simulink model "NDI"  (R2022a)
settings: Solver=ode4  StartTime=0  StopTime=100  FixedStep=fcs.Ts  RelTol=1e-3
undefined symbols (not defined in the file or in its folder): Aactuator, ac, AeroCoeff, ControlAllocation, DUmax, DUmin, EngineTable, F, fcs, ft, g, hground, IC, kg, LandingGear, Light, m, MIL, Mode_deflection_aileron, Mode_deflection_elevator, Mode_deflection_rudder, Mode_deflection_TVC_y, Mode_deflection_TVC_z, N, Ninv_2nozzle, Ninv_no_nozzle, PIController, s, Sensor, sigbuilder_block, slug, state0, sysID_DAQ, sysID_OBES, Umax_2nozzle, Umax_no_nozzle, Umin_2nozzle, Umin_no_nozzle, WMM2020
libraries: aerolibconvert2 x31, slpidlib x11, simulink x6, sharedutil x4, aerolibatmos2 x3, aerolibwind2 x3, aerolibbdyn x3, aerolibgravity2 x2, sharedtransform x1
(part 2 of 13)

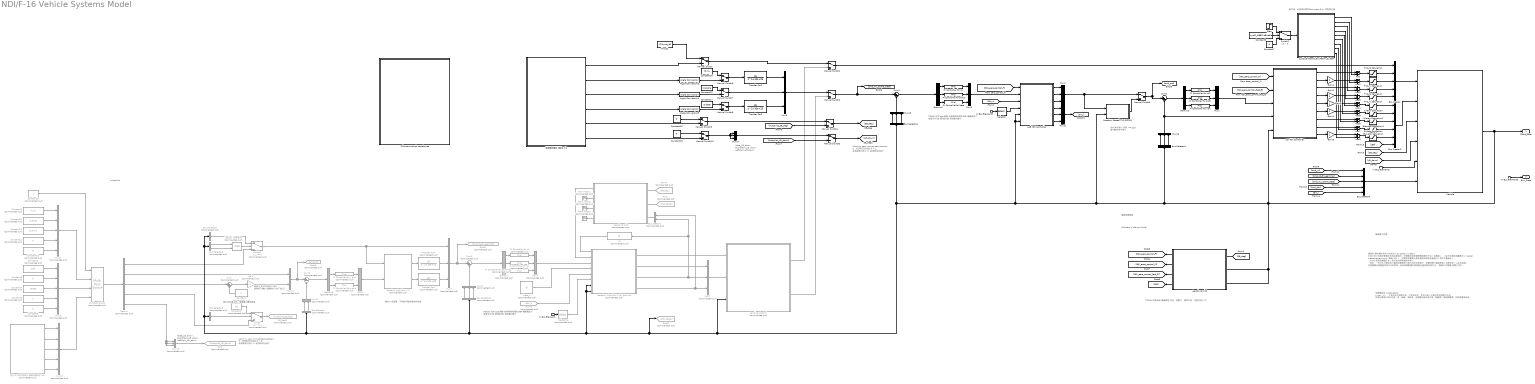
== system NDI/F-16 Vehicle Systems Model ==
  note: Onboard Airframe Model
  note: 高度 h_ft 命令是向上為正，
      | 要再乘-1轉成z座標命令(向下為正)
  note: Nose_LG_down
      | RightMain_LG_down
      | LeftMain_LG_down
  note: TODO: 改成local變數
      | 或者應該新增為OBM機載模型!?
      | 或者空中NDI跟地面NDI控制器分離!?
  note: 用於落地滑行
      | 速度 <= 220 會判斷為落地滑行
  note: 機載電子設備
  note: 全靜壓系統（pitot-static system），又稱為皮托靜壓系統、空速管系統，是飛行器上收集全壓與靜壓的系統，
      | 用來計算飛行時的空速、馬赫數、海拔等。全靜壓系統由皮托管、靜壓源、備用靜壓源、加熱裝置等組成。
  note: 傳統的 慣性導航系統(inertial navigation system (INS))至少包括計算機及含有加速度計、陀螺儀或其他運動傳感器的平台（或模組）。
      | INS包含慣性測量單元（Inertial measurement unit，簡稱 IMU ），該慣性測量單元具有角度和線性加速度計（用於位置變化）；
      | 一些IMU包括陀螺儀元件（用於保持絕對角度參考）。
      | 一般的，一個IMU內會裝有三軸的陀螺儀和三個方向的加速度計，測量物體三軸姿態角（或角速率）以及加速度。
      |
      | 在飛機顯示裝置變得現代化的同時，為其採集數據的感測器也變得更為現代化。
      | 傳統的 陀螺儀 被電子式的 航向姿態基準系統 （AHRS）與 大氣數據計算機 （ADC）所取代，
      | 在增加可靠性的同時也降低了成本、簡化了維護。
      | 此外， GPS 接收器也被整合進了玻璃駕駛艙之中。
  note: Landing gear normalized position
      | 0 : 起落架完全收起
      | 0 ~ 1: 起落架部分放下
      | 1: 起落架完全放下
  note: 拿掉!?
      | 先留著，不然配平點容易控制失敗
  note: 靜止在跑道上時，機身重心離地高度
  note: Autopilot
  note: Landing gear normalized position.
      | 0 : 起落架完全收起
      | 0 ~ 1: 起落架部分放下
      | 1: 起落架完全放下
  note: Nose_LG_down
      | RightMain_LG_down
      | LeftMain_LG_down
  note: TODO: 改成local變數
      | 或者應該新增為OBM機載模型!?
      | 或者空中NDI跟地面NDI控制器分離!?
  note: TODO: 改稱OBM機載模型
      | 內含：氣動力、標準大氣、地面作用力(?)
  note: 機載飛機模型
  note: 配平時，必須將此模塊Comment Out，否則會出錯
  In Bus Element1 : Inport  PortName=EnvData
  In Bus Element3 : Inport  PortName=EnvData
  In Bus Element2 : Inport  PortName=EnvData  Element=g
  In Bus Element : Inport  PortName=EnvData  Element=g
  Add{,1..8} (9 alike) : Sum
  Aerodynamic1 : Subsystem
  Aerodynamic2 : Subsystem  Commented=on
  Aileron Saturation : Saturate  UpperLimit=Aactuator.aileron.AngleLimitUpper  LowerLimit=Aactuator.aileron.AngleLimitLower
  Aileron Saturation1 : Saturate  UpperLimit=Aactuator.aileron.AngleLimitUpper  LowerLimit=Aactuator.aileron.AngleLimitLower
  Angle Conversion3 : aerolibconvert2/Angle Conversion  IU=deg  OU=rad
  Angle Conversion4 : aerolibconvert2/Angle Conversion  IU=deg  OU=rad
  Angle Conversion5 : aerolibconvert2/Angle Conversion  IU=deg  OU=rad
  Bus Creator : BusCreator  Inputs=5
  Bus Creator1 : BusCreator  Commented=on  Inputs=2
  Bus Creator2 : BusCreator  Inputs=6
  Bus Creator3 : BusCreator  Inputs=5
  Bus Selector : BusSelector  Commented=on  OutputSignals=epos,altitude
  Bus Selector1 : BusSelector  OutputSignals=p,q,r
  Bus Selector2 : BusSelector  Commented=on  OutputSignals=Vt
  Bus Selector3 : BusSelector  Commented=on  OutputSignals=Vt,chi,gamma
  Bus Selector4 : BusSelector  OutputSignals=mu,alpha,beta
  Bus Selector5 : BusSelector  Commented=on  OutputSignals=LGBus.Nose_WOW
  Bus Selector6 : BusSelector  Commented=on  OutputSignals=LGBus.RightMain_WOW,LGBus.LeftMain_WOW
  Constant{,3,5..6,12..13} (6 alike) : Constant  Commented=on  Value=0
  Constant1 : Constant  Commented=on  Value=60
  Constant10 : Constant  Commented=on  Value=IC.epos
  Constant11 : Constant  Commented=on  Value=IC.alt*-1
  Constant14 : Constant  Commented=on
  Constant15 : Constant  Value=IC.alpha
  Constant16 : Constant  Value=IC.mu
  Constant17 : Constant  Value=IC.beta
  Constant18 : Constant  Value=0
  Constant19 : Constant  Value=0
  Constant2 : Constant  Commented=on  Value=450
  Constant4 : Constant  Commented=on  Value=10000
  Constant7 : Constant  Value=0
  Constant8 : Constant  Value=sysID_OBES.isEnable
  Constant9 : Constant  Commented=on  Value=IC.Vt
  Demux : Demux  Commented=on  Outputs=5
  Demux1 : Demux  Commented=on  Outputs=3
  Demux3 : Demux  Outputs=3
  Demux5 : Demux  Commented=on  Outputs=2
  Demux6 : Demux  Outputs=3
  Elevator Saturation : Saturate  UpperLimit=Aactuator.elevator.AngleLimitUpper  LowerLimit=Aactuator.elevator.AngleLimitLower
  Elevator Saturation1 : Saturate  UpperLimit=Aactuator.elevator.AngleLimitUpper  LowerLimit=Aactuator.elevator.AngleLimitLower
  From : From  Commented=on  GotoTag=PlantData
  From4 : From  Commented=on  GotoTag=SB_deg
  From5 : From  Commented=on  GotoTag=LGxyz  TagVisibility=global
      settings: CloseFcn=tagdialog Close
  Gain : Gain  Commented=on  Gain=-1
  Gain{1..5} (5 alike) : Gain
  Goto : Goto  Commented=on  GotoTag=Autopilot_LG_down
  Goto1 : Goto  Commented=on  GotoTag=cmd_Vt_chi_gamma
  Goto2 : Goto  Commented=on  GotoTag=PlantData
  Goto8 : Goto  Commented=on  GotoTag=cmd_yz
  IC : InitialCondition  Commented=on  Value=IC.alpha
  Iteration Algorithm V chi gamma : Subsystem  Commented=on
  Iteration Algorithm Y Z : Subsystem  Commented=on
  Landing_Control : Subsystem  Commented=on
  Logical Operator : Logic  Commented=on  AllPortsSameDT=off  OutDataTypeStr=boolean
  Manual Switch{,1..10} (11 alike) : ManualSwitch
  Multiport Switch : MultiPortSwitch  Commented=on  SaturateOnIntegerOverflow=off  InputSameDT=off
  Mux{1..2,5..6,11,14,16,18} (8 alike) : Mux  Inputs=3
  Mux10 : Mux  Commented=on  Inputs=2
  Mux12 : Mux  Commented=on  Inputs=2
  Mux{3..4,7,13,17} (5 alike) : Mux  Commented=on  Inputs=3
  Mux15 : Mux  Commented=on  Inputs=5
  Mux19 : Mux  Commented=on  Inputs=5
  Mux8 : Mux  Commented=on  Inputs=5
  Mux9 : Mux  Commented=on  Inputs=2
  PI Controller for Vt : slpidlib/PID Controller  Commented=on  Controller=PI  Form=Parallel  TimeDomain=Continuous-time  UseExternalTs=off  SampleTime=-1  IntegratorMethod=Forward Euler  FilterMethod=Forward Euler  ControllerParametersSource=internal  P=PIController.Vt.P  I=PIController.Vt.I  UseKiTs=off  D=0  N=100  UseFilter=on  TunerSelectOption=Transfer Function Based (PID Tuner App)  InitialConditionSource=internal  InitialConditionForIntegrator=0  InitialConditionForFilter=0  DifferentiatorICPrevScaledInput=0  ExternalReset=none  TrackingMode=off  Kt=1  LimitOutput=off  SatLimitsSource=internal  UpperSaturationLimit=inf  LowerSaturationLimit=-inf  LinearizeAsGain=on  AntiWindupMode=none  Kb=1  POutMin=[]  POutMax=[]  IOutMin=[]  IOutMax=[]  DOutMin=[]  DOutMax=[]  NOutMin=[]  NOutMax=[]  SumOutMin=[]  SumOutMax=[]  SaturationOutMin=[]  SaturationOutMax=[]  PParamMin=[]  PParamMax=[]  IParamMin=[]  IParamMax=[]  DParamMin=[]  DParamMax=[]  NParamMin=[]  NParamMax=[]  KbParamMin=[]  KbParamMax=[]  KtParamMin=[]  KtParamMax=[]  KbOutMin=[]  KbOutMax=[]  KtOutMin=[]  KtOutMax=[]  IntegratorOutMin=[]  IntegratorOutMax=[]  FilterOutMin=[]  FilterOutMax=[]  SumI1OutMin=[]  SumI1OutMax=[]  SumI2OutMin=[]  SumI2OutMax=[]  SumI3OutMin=[]  SumI3OutMax=[]  SumI4OutMin=[]  SumI4OutMax=[]  SumDOutMin=[]  SumDOutMax=[]  DifferentiatorOutMin=[]  DifferentiatorOutMax=[]  FilterDiffOutCoefMin=[]  FilterDiffOutCoefMax=[]  ReciprocalOutMin=[]  ReciprocalOutMax=[]  SumDenOutMin=[]  SumDenOutMax=[]  SumNumOutMin=[]  SumNumOutMax=[]  DivideOutMin=[]  DivideOutMax=[]  UdiffTsProdOutMin=[]  UdiffTsProdOutMax=[]  NTsProdOutMin=[]  NTsProdOutMax=[]  UintegralTsProdOutMin=[]  UintegralTsProdOutMax=[]  UngainTsProdOutMin=[]  UngainTsProdOutMax=[]  IntegratorContinuousStateAttributes=''  IntegratorStateMustResolveToSignalObject=off  IntegratorRTWStateStorageClass=Auto  FilterContinuousStateAttributes=''  FilterStateMustResolveToSignalObject=off  FilterRTWStateStorageClass=Auto  ParallelPVariant=InternalParameters  IdealPVariant=Disabled  IVariant=InternalParameters  DVariant=Disabled  IntegratorVariant=Continuous  SatVariant=Disabled  AWVariant=Passthrough  PCopyVariant=Disabled  TRVariant=Disabled  FdbkBlocksVariant=Forward  IdealPFdbkVariant=Disabled  SatFdbkVariant=Disabled  DerivativeFilterVariant=Disabled  NVariant=Disabled  NCopyVariant=Disabled_SignalSpec  FilterICVariant=Disabled  IntegratorICVariant=InternalICs  ExternalResetVariant=Disabled  TRSumVariant=Passthrough  SumFdbkVariant=Disabled  SumVariant=Sum_PI  TsampFilterVariant=InternalTs  TsampNgainVariant=Passthrough  TsampIntegralVariant=Passthrough  ExternalSaturationOutDataTypeStr=Inherit: Same as second input  aMode=0
  PI Controller for alpha : slpidlib/PID Controller  Controller=PI  Form=Parallel  TimeDomain=Continuous-time  UseExternalTs=off  SampleTime=-1  IntegratorMethod=Forward Euler  FilterMethod=Forward Euler  ControllerParametersSource=internal  P=PIController.alpha.P  I=PIController.alpha.I  UseKiTs=off  D=0  N=100  UseFilter=on  TunerSelectOption=Transfer Function Based (PID Tuner App)  InitialConditionSource=internal  InitialConditionForIntegrator=0  InitialConditionForFilter=0  DifferentiatorICPrevScaledInput=0  ExternalReset=none  TrackingMode=off  Kt=1  LimitOutput=off  SatLimitsSource=internal  UpperSaturationLimit=inf  LowerSaturationLimit=-inf  LinearizeAsGain=on  AntiWindupMode=none  Kb=1  POutMin=[]  POutMax=[]  IOutMin=[]  IOutMax=[]  DOutMin=[]  DOutMax=[]  NOutMin=[]  NOutMax=[]  SumOutMin=[]  SumOutMax=[]  SaturationOutMin=[]  SaturationOutMax=[]  PParamMin=[]  PParamMax=[]  IParamMin=[]  IParamMax=[]  DParamMin=[]  DParamMax=[]  NParamMin=[]  NParamMax=[]  KbParamMin=[]  KbParamMax=[]  KtParamMin=[]  KtParamMax=[]  KbOutMin=[]  KbOutMax=[]  KtOutMin=[]  KtOutMax=[]  IntegratorOutMin=[]  IntegratorOutMax=[]  FilterOutMin=[]  FilterOutMax=[]  SumI1OutMin=[]  SumI1OutMax=[]  SumI2OutMin=[]  SumI2OutMax=[]  SumI3OutMin=[]  SumI3OutMax=[]  SumI4OutMin=[]  SumI4OutMax=[]  SumDOutMin=[]  SumDOutMax=[]  DifferentiatorOutMin=[]  DifferentiatorOutMax=[]  FilterDiffOutCoefMin=[]  FilterDiffOutCoefMax=[]  ReciprocalOutMin=[]  ReciprocalOutMax=[]  SumDenOutMin=[]  SumDenOutMax=[]  SumNumOutMin=[]  SumNumOutMax=[]  DivideOutMin=[]  DivideOutMax=[]  UdiffTsProdOutMin=[]  UdiffTsProdOutMax=[]  NTsProdOutMin=[]  NTsProdOutMax=[]  UintegralTsProdOutMin=[]  UintegralTsProdOutMax=[]  UngainTsProdOutMin=[]  UngainTsProdOutMax=[]  IntegratorContinuousStateAttributes=''  IntegratorStateMustResolveToSignalObject=off  IntegratorRTWStateStorageClass=Auto  FilterContinuousStateAttributes=''  FilterStateMustResolveToSignalObject=off  FilterRTWStateStorageClass=Auto  ParallelPVariant=InternalParameters  IdealPVariant=Disabled  IVariant=InternalParameters  DVariant=Disabled  IntegratorVariant=Continuous  SatVariant=Disabled  AWVariant=Passthrough  PCopyVariant=Disabled  TRVariant=Disabled  FdbkBlocksVariant=Forward  IdealPFdbkVariant=Disabled  SatFdbkVariant=Disabled  DerivativeFilterVariant=Disabled  NVariant=Disabled  NCopyVariant=Disabled_SignalSpec  FilterICVariant=Disabled  IntegratorICVariant=InternalICs  ExternalResetVariant=Disabled  TRSumVariant=Passthrough  SumFdbkVariant=Disabled  SumVariant=Sum_PI  TsampFilterVariant=InternalTs  TsampNgainVariant=Passthrough  TsampIntegralVariant=Passthrough  ExternalSaturationOutDataTypeStr=Inherit: Same as second input  aMode=0
  PI Controller for beta : slpidlib/PID Controller  Controller=PI  Form=Parallel  TimeDomain=Continuous-time  UseExternalTs=off  SampleTime=-1  IntegratorMethod=Forward Euler  FilterMethod=Forward Euler  ControllerParametersSource=internal  P=PIController.beta.P  I=PIController.beta.I  UseKiTs=off  D=0  N=100  UseFilter=on  TunerSelectOption=Transfer Function Based (PID Tuner App)  InitialConditionSource=internal  InitialConditionForIntegrator=0  InitialConditionForFilter=0  DifferentiatorICPrevScaledInput=0  ExternalReset=none  TrackingMode=off  Kt=1  LimitOutput=off  SatLimitsSource=internal  UpperSaturationLimit=inf  LowerSaturationLimit=-inf  LinearizeAsGain=on  AntiWindupMode=none  Kb=1  POutMin=[]  POutMax=[]  IOutMin=[]  IOutMax=[]  DOutMin=[]  DOutMax=[]  NOutMin=[]  NOutMax=[]  SumOutMin=[]  SumOutMax=[]  SaturationOutMin=[]  SaturationOutMax=[]  PParamMin=[]  PParamMax=[]  IParamMin=[]  IParamMax=[]  DParamMin=[]  DParamMax=[]  NParamMin=[]  NParamMax=[]  KbParamMin=[]  KbParamMax=[]  KtParamMin=[]  KtParamMax=[]  KbOutMin=[]  KbOutMax=[]  KtOutMin=[]  KtOutMax=[]  IntegratorOutMin=[]  IntegratorOutMax=[]  FilterOutMin=[]  FilterOutMax=[]  SumI1OutMin=[]  SumI1OutMax=[]  SumI2OutMin=[]  SumI2OutMax=[]  SumI3OutMin=[]  SumI3OutMax=[]  SumI4OutMin=[]  SumI4OutMax=[]  SumDOutMin=[]  SumDOutMax=[]  DifferentiatorOutMin=[]  DifferentiatorOutMax=[]  FilterDiffOutCoefMin=[]  FilterDiffOutCoefMax=[]  ReciprocalOutMin=[]  ReciprocalOutMax=[]  SumDenOutMin=[]  SumDenOutMax=[]  SumNumOutMin=[]  SumNumOutMax=[]  DivideOutMin=[]  DivideOutMax=[]  UdiffTsProdOutMin=[]  UdiffTsProdOutMax=[]  NTsProdOutMin=[]  NTsProdOutMax=[]  UintegralTsProdOutMin=[]  UintegralTsProdOutMax=[]  UngainTsProdOutMin=[]  UngainTsProdOutMax=[]  IntegratorContinuousStateAttributes=''  IntegratorStateMustResolveToSignalObject=off  IntegratorRTWStateStorageClass=Auto  FilterContinuousStateAttributes=''  FilterStateMustResolveToSignalObject=off  FilterRTWStateStorageClass=Auto  ParallelPVariant=InternalParameters  IdealPVariant=Disabled  IVariant=InternalParameters  DVariant=Disabled  IntegratorVariant=Continuous  SatVariant=Disabled  AWVariant=Passthrough  PCopyVariant=Disabled  TRVariant=Disabled  FdbkBlocksVariant=Forward  IdealPFdbkVariant=Disabled  SatFdbkVariant=Disabled  DerivativeFilterVariant=Disabled  NVariant=Disabled  NCopyVariant=Disabled_SignalSpec  FilterICVariant=Disabled  IntegratorICVariant=InternalICs  ExternalResetVariant=Disabled  TRSumVariant=Passthrough  SumFdbkVariant=Disabled  SumVariant=Sum_PI  TsampFilterVariant=InternalTs  TsampNgainVariant=Passthrough  TsampIntegralVariant=Passthrough  ExternalSaturationOutDataTypeStr=Inherit: Same as second input  aMode=0
  PI Controller for chi : slpidlib/PID Controller  Commented=on  Controller=PI  Form=Parallel  TimeDomain=Continuous-time  UseExternalTs=off  SampleTime=-1  IntegratorMethod=Forward Euler  FilterMethod=Forward Euler  ControllerParametersSource=internal  P=PIController.chi.P  I=PIController.chi.I  UseKiTs=off  D=0  N=100  UseFilter=on  TunerSelectOption=Transfer Function Based (PID Tuner App)  InitialConditionSource=internal  InitialConditionForIntegrator=0  InitialConditionForFilter=0  DifferentiatorICPrevScaledInput=0  ExternalReset=none  TrackingMode=off  Kt=1  LimitOutput=off  SatLimitsSource=internal  UpperSaturationLimit=inf  LowerSaturationLimit=-inf  LinearizeAsGain=on  AntiWindupMode=none  Kb=1  POutMin=[]  POutMax=[]  IOutMin=[]  IOutMax=[]  DOutMin=[]  DOutMax=[]  NOutMin=[]  NOutMax=[]  SumOutMin=[]  SumOutMax=[]  SaturationOutMin=[]  SaturationOutMax=[]  PParamMin=[]  PParamMax=[]  IParamMin=[]  IParamMax=[]  DParamMin=[]  DParamMax=[]  NParamMin=[]  NParamMax=[]  KbParamMin=[]  KbParamMax=[]  KtParamMin=[]  KtParamMax=[]  KbOutMin=[]  KbOutMax=[]  KtOutMin=[]  KtOutMax=[]  IntegratorOutMin=[]  IntegratorOutMax=[]  FilterOutMin=[]  FilterOutMax=[]  SumI1OutMin=[]  SumI1OutMax=[]  SumI2OutMin=[]  SumI2OutMax=[]  SumI3OutMin=[]  SumI3OutMax=[]  SumI4OutMin=[]  SumI4OutMax=[]  SumDOutMin=[]  SumDOutMax=[]  DifferentiatorOutMin=[]  DifferentiatorOutMax=[]  FilterDiffOutCoefMin=[]  FilterDiffOutCoefMax=[]  ReciprocalOutMin=[]  ReciprocalOutMax=[]  SumDenOutMin=[]  SumDenOutMax=[]  SumNumOutMin=[]  SumNumOutMax=[]  DivideOutMin=[]  DivideOutMax=[]  UdiffTsProdOutMin=[]  UdiffTsProdOutMax=[]  NTsProdOutMin=[]  NTsProdOutMax=[]  UintegralTsProdOutMin=[]  UintegralTsProdOutMax=[]  UngainTsProdOutMin=[]  UngainTsProdOutMax=[]  IntegratorContinuousStateAttributes=''  IntegratorStateMustResolveToSignalObject=off  IntegratorRTWStateStorageClass=Auto  FilterContinuousStateAttributes=''  FilterStateMustResolveToSignalObject=off  FilterRTWStateStorageClass=Auto  ParallelPVariant=InternalParameters  IdealPVariant=Disabled  IVariant=InternalParameters  DVariant=Disabled  IntegratorVariant=Continuous  SatVariant=Disabled  AWVariant=Passthrough  PCopyVariant=Disabled  TRVariant=Disabled  FdbkBlocksVariant=Forward  IdealPFdbkVariant=Disabled  SatFdbkVariant=Disabled  DerivativeFilterVariant=Disabled  NVariant=Disabled  NCopyVariant=Disabled_SignalSpec  FilterICVariant=Disabled  IntegratorICVariant=InternalICs  ExternalResetVariant=Disabled  TRSumVariant=Passthrough  SumFdbkVariant=Disabled  SumVariant=Sum_PI  TsampFilterVariant=InternalTs  TsampNgainVariant=Passthrough  TsampIntegralVariant=Passthrough  ExternalSaturationOutDataTypeStr=Inherit: Same as second input  aMode=0
  PI Controller for gamma : slpidlib/PID Controller  Commented=on  Controller=PI  Form=Parallel  TimeDomain=Continuous-time  UseExternalTs=off  SampleTime=-1  IntegratorMethod=Forward Euler  FilterMethod=Forward Euler  ControllerParametersSource=internal  P=PIController.gamma.P  I=PIController.gamma.I  UseKiTs=off  D=0  N=100  UseFilter=on  TunerSelectOption=Transfer Function Based (PID Tuner App)  InitialConditionSource=internal  InitialConditionForIntegrator=0  InitialConditionForFilter=0  DifferentiatorICPrevScaledInput=0  ExternalReset=none  TrackingMode=off  Kt=1  LimitOutput=off  SatLimitsSource=internal  UpperSaturationLimit=inf  LowerSaturationLimit=-inf  LinearizeAsGain=on  AntiWindupMode=none  Kb=1  POutMin=[]  POutMax=[]  IOutMin=[]  IOutMax=[]  DOutMin=[]  DOutMax=[]  NOutMin=[]  NOutMax=[]  SumOutMin=[]  SumOutMax=[]  SaturationOutMin=[]  SaturationOutMax=[]  PParamMin=[]  PParamMax=[]  IParamMin=[]  IParamMax=[]  DParamMin=[]  DParamMax=[]  NParamMin=[]  NParamMax=[]  KbParamMin=[]  KbParamMax=[]  KtParamMin=[]  KtParamMax=[]  KbOutMin=[]  KbOutMax=[]  KtOutMin=[]  KtOutMax=[]  IntegratorOutMin=[]  IntegratorOutMax=[]  FilterOutMin=[]  FilterOutMax=[]  SumI1OutMin=[]  SumI1OutMax=[]  SumI2OutMin=[]  SumI2OutMax=[]  SumI3OutMin=[]  SumI3OutMax=[]  SumI4OutMin=[]  SumI4OutMax=[]  SumDOutMin=[]  SumDOutMax=[]  DifferentiatorOutMin=[]  DifferentiatorOutMax=[]  FilterDiffOutCoefMin=[]  FilterDiffOutCoefMax=[]  ReciprocalOutMin=[]  ReciprocalOutMax=[]  SumDenOutMin=[]  SumDenOutMax=[]  SumNumOutMin=[]  SumNumOutMax=[]  DivideOutMin=[]  DivideOutMax=[]  UdiffTsProdOutMin=[]  UdiffTsProdOutMax=[]  NTsProdOutMin=[]  NTsProdOutMax=[]  UintegralTsProdOutMin=[]  UintegralTsProdOutMax=[]  UngainTsProdOutMin=[]  UngainTsProdOutMax=[]  IntegratorContinuousStateAttributes=''  IntegratorStateMustResolveToSignalObject=off  IntegratorRTWStateStorageClass=Auto  FilterContinuousStateAttributes=''  FilterStateMustResolveToSignalObject=off  FilterRTWStateStorageClass=Auto  ParallelPVariant=InternalParameters  IdealPVariant=Disabled  IVariant=InternalParameters  DVariant=Disabled  IntegratorVariant=Continuous  SatVariant=Disabled  AWVariant=Passthrough  PCopyVariant=Disabled  TRVariant=Disabled  FdbkBlocksVariant=Forward  IdealPFdbkVariant=Disabled  SatFdbkVariant=Disabled  DerivativeFilterVariant=Disabled  NVariant=Disabled  NCopyVariant=Disabled_SignalSpec  FilterICVariant=Disabled  IntegratorICVariant=InternalICs  ExternalResetVariant=Disabled  TRSumVariant=Passthrough  SumFdbkVariant=Disabled  SumVariant=Sum_PI  TsampFilterVariant=InternalTs  TsampNgainVariant=Passthrough  TsampIntegralVariant=Passthrough  ExternalSaturationOutDataTypeStr=Inherit: Same as second input  aMode=0
  PI Controller for mu : slpidlib/PID Controller  Controller=PI  Form=Parallel  TimeDomain=Continuous-time  UseExternalTs=off  SampleTime=-1  IntegratorMethod=Forward Euler  FilterMethod=Forward Euler  ControllerParametersSource=internal  P=PIController.mu.P  I=PIController.mu.I  UseKiTs=off  D=0  N=100  UseFilter=on  TunerSelectOption=Transfer Function Based (PID Tuner App)  InitialConditionSource=internal  InitialConditionForIntegrator=0  InitialConditionForFilter=0  DifferentiatorICPrevScaledInput=0  ExternalReset=none  TrackingMode=off  Kt=1  LimitOutput=off  SatLimitsSource=internal  UpperSaturationLimit=inf  LowerSaturationLimit=-inf  LinearizeAsGain=on  AntiWindupMode=none  Kb=1  POutMin=[]  POutMax=[]  IOutMin=[]  IOutMax=[]  DOutMin=[]  DOutMax=[]  NOutMin=[]  NOutMax=[]  SumOutMin=[]  SumOutMax=[]  SaturationOutMin=[]  SaturationOutMax=[]  PParamMin=[]  PParamMax=[]  IParamMin=[]  IParamMax=[]  DParamMin=[]  DParamMax=[]  NParamMin=[]  NParamMax=[]  KbParamMin=[]  KbParamMax=[]  KtParamMin=[]  KtParamMax=[]  KbOutMin=[]  KbOutMax=[]  KtOutMin=[]  KtOutMax=[]  IntegratorOutMin=[]  IntegratorOutMax=[]  FilterOutMin=[]  FilterOutMax=[]  SumI1OutMin=[]  SumI1OutMax=[]  SumI2OutMin=[]  SumI2OutMax=[]  SumI3OutMin=[]  SumI3OutMax=[]  SumI4OutMin=[]  SumI4OutMax=[]  SumDOutMin=[]  SumDOutMax=[]  DifferentiatorOutMin=[]  DifferentiatorOutMax=[]  FilterDiffOutCoefMin=[]  FilterDiffOutCoefMax=[]  ReciprocalOutMin=[]  ReciprocalOutMax=[]  SumDenOutMin=[]  SumDenOutMax=[]  SumNumOutMin=[]  SumNumOutMax=[]  DivideOutMin=[]  DivideOutMax=[]  UdiffTsProdOutMin=[]  UdiffTsProdOutMax=[]  NTsProdOutMin=[]  NTsProdOutMax=[]  UintegralTsProdOutMin=[]  UintegralTsProdOutMax=[]  UngainTsProdOutMin=[]  UngainTsProdOutMax=[]  IntegratorContinuousStateAttributes=''  IntegratorStateMustResolveToSignalObject=off  IntegratorRTWStateStorageClass=Auto  FilterContinuousStateAttributes=''  FilterStateMustResolveToSignalObject=off  FilterRTWStateStorageClass=Auto  ParallelPVariant=InternalParameters  IdealPVariant=Disabled  IVariant=InternalParameters  DVariant=Disabled  IntegratorVariant=Continuous  SatVariant=Disabled  AWVariant=Passthrough  PCopyVariant=Disabled  TRVariant=Disabled  FdbkBlocksVariant=Forward  IdealPFdbkVariant=Disabled  SatFdbkVariant=Disabled  DerivativeFilterVariant=Disabled  NVariant=Disabled  NCopyVariant=Disabled_SignalSpec  FilterICVariant=Disabled  IntegratorICVariant=InternalICs  ExternalResetVariant=Disabled  TRSumVariant=Passthrough  SumFdbkVariant=Disabled  SumVariant=Sum_PI  TsampFilterVariant=InternalTs  TsampNgainVariant=Passthrough  TsampIntegralVariant=Passthrough  ExternalSaturationOutDataTypeStr=Inherit: Same as second input  aMode=0
  PI Controller for pitch : slpidlib/PID Controller  Controller=PI  Form=Parallel  TimeDomain=Continuous-time  UseExternalTs=off  SampleTime=-1  IntegratorMethod=Forward Euler  FilterMethod=Forward Euler  ControllerParametersSource=internal  P=PIController.q.P  I=PIController.q.I  UseKiTs=off  D=0  N=100  UseFilter=on  TunerSelectOption=Transfer Function Based (PID Tuner App)  InitialConditionSource=internal  InitialConditionForIntegrator=0  InitialConditionForFilter=0  DifferentiatorICPrevScaledInput=0  ExternalReset=none  TrackingMode=off  Kt=1  LimitOutput=off  SatLimitsSource=internal  UpperSaturationLimit=inf  LowerSaturationLimit=-inf  LinearizeAsGain=on  AntiWindupMode=none  Kb=1  POutMin=[]  POutMax=[]  IOutMin=[]  IOutMax=[]  DOutMin=[]  DOutMax=[]  NOutMin=[]  NOutMax=[]  SumOutMin=[]  SumOutMax=[]  SaturationOutMin=[]  SaturationOutMax=[]  PParamMin=[]  PParamMax=[]  IParamMin=[]  IParamMax=[]  DParamMin=[]  DParamMax=[]  NParamMin=[]  NParamMax=[]  KbParamMin=[]  KbParamMax=[]  KtParamMin=[]  KtParamMax=[]  KbOutMin=[]  KbOutMax=[]  KtOutMin=[]  KtOutMax=[]  IntegratorOutMin=[]  IntegratorOutMax=[]  FilterOutMin=[]  FilterOutMax=[]  SumI1OutMin=[]  SumI1OutMax=[]  SumI2OutMin=[]  SumI2OutMax=[]  SumI3OutMin=[]  SumI3OutMax=[]  SumI4OutMin=[]  SumI4OutMax=[]  SumDOutMin=[]  SumDOutMax=[]  DifferentiatorOutMin=[]  DifferentiatorOutMax=[]  FilterDiffOutCoefMin=[]  FilterDiffOutCoefMax=[]  ReciprocalOutMin=[]  ReciprocalOutMax=[]  SumDenOutMin=[]  SumDenOutMax=[]  SumNumOutMin=[]  SumNumOutMax=[]  DivideOutMin=[]  DivideOutMax=[]  UdiffTsProdOutMin=[]  UdiffTsProdOutMax=[]  NTsProdOutMin=[]  NTsProdOutMax=[]  UintegralTsProdOutMin=[]  UintegralTsProdOutMax=[]  UngainTsProdOutMin=[]  UngainTsProdOutMax=[]  IntegratorContinuousStateAttributes=''  IntegratorStateMustResolveToSignalObject=off  IntegratorRTWStateStorageClass=Auto  FilterContinuousStateAttributes=''  FilterStateMustResolveToSignalObject=off  FilterRTWStateStorageClass=Auto  ParallelPVariant=InternalParameters  IdealPVariant=Disabled  IVariant=InternalParameters  DVariant=Disabled  IntegratorVariant=Continuous  SatVariant=Disabled  AWVariant=Passthrough  PCopyVariant=Disabled  TRVariant=Disabled  FdbkBlocksVariant=Forward  IdealPFdbkVariant=Disabled  SatFdbkVariant=Disabled  DerivativeFilterVariant=Disabled  NVariant=Disabled  NCopyVariant=Disabled_SignalSpec  FilterICVariant=Disabled  IntegratorICVariant=InternalICs  ExternalResetVariant=Disabled  TRSumVariant=Passthrough  SumFdbkVariant=Disabled  SumVariant=Sum_PI  TsampFilterVariant=InternalTs  TsampNgainVariant=Passthrough  TsampIntegralVariant=Passthrough  ExternalSaturationOutDataTypeStr=Inherit: Same as second input  aMode=0
  PI Controller for roll : slpidlib/PID Controller  Controller=PI  Form=Parallel  TimeDomain=Continuous-time  UseExternalTs=off  SampleTime=-1  IntegratorMethod=Forward Euler  FilterMethod=Forward Euler  ControllerParametersSource=internal  P=PIController.p.P  I=PIController.p.I  UseKiTs=off  D=0  N=100  UseFilter=on  TunerSelectOption=Transfer Function Based (PID Tuner App)  InitialConditionSource=internal  InitialConditionForIntegrator=0  InitialConditionForFilter=0  DifferentiatorICPrevScaledInput=0  ExternalReset=none  TrackingMode=off  Kt=1  LimitOutput=off  SatLimitsSource=internal  UpperSaturationLimit=inf  LowerSaturationLimit=-inf  LinearizeAsGain=on  AntiWindupMode=none  Kb=1  POutMin=[]  POutMax=[]  IOutMin=[]  IOutMax=[]  DOutMin=[]  DOutMax=[]  NOutMin=[]  NOutMax=[]  SumOutMin=[]  SumOutMax=[]  SaturationOutMin=[]  SaturationOutMax=[]  PParamMin=[]  PParamMax=[]  IParamMin=[]  IParamMax=[]  DParamMin=[]  DParamMax=[]  NParamMin=[]  NParamMax=[]  KbParamMin=[]  KbParamMax=[]  KtParamMin=[]  KtParamMax=[]  KbOutMin=[]  KbOutMax=[]  KtOutMin=[]  KtOutMax=[]  IntegratorOutMin=[]  IntegratorOutMax=[]  FilterOutMin=[]  FilterOutMax=[]  SumI1OutMin=[]  SumI1OutMax=[]  SumI2OutMin=[]  SumI2OutMax=[]  SumI3OutMin=[]  SumI3OutMax=[]  SumI4OutMin=[]  SumI4OutMax=[]  SumDOutMin=[]  SumDOutMax=[]  DifferentiatorOutMin=[]  DifferentiatorOutMax=[]  FilterDiffOutCoefMin=[]  FilterDiffOutCoefMax=[]  ReciprocalOutMin=[]  ReciprocalOutMax=[]  SumDenOutMin=[]  SumDenOutMax=[]  SumNumOutMin=[]  SumNumOutMax=[]  DivideOutMin=[]  DivideOutMax=[]  UdiffTsProdOutMin=[]  UdiffTsProdOutMax=[]  NTsProdOutMin=[]  NTsProdOutMax=[]  UintegralTsProdOutMin=[]  UintegralTsProdOutMax=[]  UngainTsProdOutMin=[]  UngainTsProdOutMax=[]  IntegratorContinuousStateAttributes=''  IntegratorStateMustResolveToSignalObject=off  IntegratorRTWStateStorageClass=Auto  FilterContinuousStateAttributes=''  FilterStateMustResolveToSignalObject=off  FilterRTWStateStorageClass=Auto  ParallelPVariant=InternalParameters  IdealPVariant=Disabled  IVariant=InternalParameters  DVariant=Disabled  IntegratorVariant=Continuous  SatVariant=Disabled  AWVariant=Passthrough  PCopyVariant=Disabled  TRVariant=Disabled  FdbkBlocksVariant=Forward  IdealPFdbkVariant=Disabled  SatFdbkVariant=Disabled  DerivativeFilterVariant=Disabled  NVariant=Disabled  NCopyVariant=Disabled_SignalSpec  FilterICVariant=Disabled  IntegratorICVariant=InternalICs  ExternalResetVariant=Disabled  TRSumVariant=Passthrough  SumFdbkVariant=Disabled  SumVariant=Sum_PI  TsampFilterVariant=InternalTs  TsampNgainVariant=Passthrough  TsampIntegralVariant=Passthrough  ExternalSaturationOutDataTypeStr=Inherit: Same as second input  aMode=0
  PI Controller for y axis : slpidlib/PID Controller  Commented=on  Controller=PI  Form=Parallel  TimeDomain=Continuous-time  UseExternalTs=off  SampleTime=-1  IntegratorMethod=Forward Euler  FilterMethod=Forward Euler  ControllerParametersSource=internal  P=PIController.y.P  I=PIController.y.I  UseKiTs=off  D=PIController.y.D  N=10  UseFilter=on  TunerSelectOption=Transfer Function Based (PID Tuner App)  InitialConditionSource=internal  InitialConditionForIntegrator=0  InitialConditionForFilter=0  DifferentiatorICPrevScaledInput=0  ExternalReset=none  TrackingMode=off  Kt=1  LimitOutput=off  SatLimitsSource=internal  UpperSaturationLimit=inf  LowerSaturationLimit=-inf  LinearizeAsGain=on  AntiWindupMode=none  Kb=1  POutMin=[]  POutMax=[]  IOutMin=[]  IOutMax=[]  DOutMin=[]  DOutMax=[]  NOutMin=[]  NOutMax=[]  SumOutMin=[]  SumOutMax=[]  SaturationOutMin=[]  SaturationOutMax=[]  PParamMin=[]  PParamMax=[]  IParamMin=[]  IParamMax=[]  DParamMin=[]  DParamMax=[]  NParamMin=[]  NParamMax=[]  KbParamMin=[]  KbParamMax=[]  KtParamMin=[]  KtParamMax=[]  KbOutMin=[]  KbOutMax=[]  KtOutMin=[]  KtOutMax=[]  IntegratorOutMin=[]  IntegratorOutMax=[]  FilterOutMin=[]  FilterOutMax=[]  SumI1OutMin=[]  SumI1OutMax=[]  SumI2OutMin=[]  SumI2OutMax=[]  SumI3OutMin=[]  SumI3OutMax=[]  SumI4OutMin=[]  SumI4OutMax=[]  SumDOutMin=[]  SumDOutMax=[]  DifferentiatorOutMin=[]  DifferentiatorOutMax=[]  FilterDiffOutCoefMin=[]  FilterDiffOutCoefMax=[]  ReciprocalOutMin=[]  ReciprocalOutMax=[]  SumDenOutMin=[]  SumDenOutMax=[]  SumNumOutMin=[]  SumNumOutMax=[]  DivideOutMin=[]  DivideOutMax=[]  UdiffTsProdOutMin=[]  UdiffTsProdOutMax=[]  NTsProdOutMin=[]  NTsProdOutMax=[]  UintegralTsProdOutMin=[]  UintegralTsProdOutMax=[]  UngainTsProdOutMin=[]  UngainTsProdOutMax=[]  IntegratorContinuousStateAttributes=''  IntegratorStateMustResolveToSignalObject=off  IntegratorRTWStateStorageClass=Auto  FilterContinuousStateAttributes=''  FilterStateMustResolveToSignalObject=off  FilterRTWStateStorageClass=Auto  ParallelPVariant=InternalParameters  IdealPVariant=Disabled  IVariant=InternalParameters  DVariant=Disabled  IntegratorVariant=Continuous  SatVariant=Disabled  AWVariant=Passthrough  PCopyVariant=Disabled  TRVariant=Disabled  FdbkBlocksVariant=Forward  IdealPFdbkVariant=Disabled  SatFdbkVariant=Disabled  DerivativeFilterVariant=Disabled  NVariant=Disabled  NCopyVariant=Disabled_SignalSpec  FilterICVariant=Disabled  IntegratorICVariant=InternalICs  ExternalResetVariant=Disabled  TRSumVariant=Passthrough  SumFdbkVariant=Disabled  SumVariant=Sum_PI  TsampFilterVariant=InternalTs  TsampNgainVariant=Passthrough  TsampIntegralVariant=Passthrough  ExternalSaturationOutDataTypeStr=Inherit: Same as second input  aMode=0
  PI Controller for yaw : slpidlib/PID Controller  Controller=PI  Form=Parallel  TimeDomain=Continuous-time  UseExternalTs=off  SampleTime=-1  IntegratorMethod=Forward Euler  FilterMethod=Forward Euler  ControllerParametersSource=internal  P=PIController.r.P  I=PIController.r.I  UseKiTs=off  D=0  N=100  UseFilter=on  TunerSelectOption=Transfer Function Based (PID Tuner App)  InitialConditionSource=internal  InitialConditionForIntegrator=0  InitialConditionForFilter=0  DifferentiatorICPrevScaledInput=0  ExternalReset=none  TrackingMode=off  Kt=1  LimitOutput=off  SatLimitsSource=internal  UpperSaturationLimit=inf  LowerSaturationLimit=-inf  LinearizeAsGain=on  AntiWindupMode=none  Kb=1  POutMin=[]  POutMax=[]  IOutMin=[]  IOutMax=[]  DOutMin=[]  DOutMax=[]  NOutMin=[]  NOutMax=[]  SumOutMin=[]  SumOutMax=[]  SaturationOutMin=[]  SaturationOutMax=[]  PParamMin=[]  PParamMax=[]  IParamMin=[]  IParamMax=[]  DParamMin=[]  DParamMax=[]  NParamMin=[]  NParamMax=[]  KbParamMin=[]  KbParamMax=[]  KtParamMin=[]  KtParamMax=[]  KbOutMin=[]  KbOutMax=[]  KtOutMin=[]  KtOutMax=[]  IntegratorOutMin=[]  IntegratorOutMax=[]  FilterOutMin=[]  FilterOutMax=[]  SumI1OutMin=[]  SumI1OutMax=[]  SumI2OutMin=[]  SumI2OutMax=[]  SumI3OutMin=[]  SumI3OutMax=[]  SumI4OutMin=[]  SumI4OutMax=[]  SumDOutMin=[]  SumDOutMax=[]  DifferentiatorOutMin=[]  DifferentiatorOutMax=[]  FilterDiffOutCoefMin=[]  FilterDiffOutCoefMax=[]  ReciprocalOutMin=[]  ReciprocalOutMax=[]  SumDenOutMin=[]  SumDenOutMax=[]  SumNumOutMin=[]  SumNumOutMax=[]  DivideOutMin=[]  DivideOutMax=[]  UdiffTsProdOutMin=[]  UdiffTsProdOutMax=[]  NTsProdOutMin=[]  NTsProdOutMax=[]  UintegralTsProdOutMin=[]  UintegralTsProdOutMax=[]  UngainTsProdOutMin=[]  UngainTsProdOutMax=[]  IntegratorContinuousStateAttributes=''  IntegratorStateMustResolveToSignalObject=off  IntegratorRTWStateStorageClass=Auto  FilterContinuousStateAttributes=''  FilterStateMustResolveToSignalObject=off  FilterRTWStateStorageClass=Auto  ParallelPVariant=InternalParameters  IdealPVariant=Disabled  IVariant=InternalParameters  DVariant=Disabled  IntegratorVariant=Continuous  SatVariant=Disabled  AWVariant=Passthrough  PCopyVariant=Disabled  TRVariant=Disabled  FdbkBlocksVariant=Forward  IdealPFdbkVariant=Disabled  SatFdbkVariant=Disabled  DerivativeFilterVariant=Disabled  NVariant=Disabled  NCopyVariant=Disabled_SignalSpec  FilterICVariant=Disabled  IntegratorICVariant=InternalICs  ExternalResetVariant=Disabled  TRSumVariant=Passthrough  SumFdbkVariant=Disabled  SumVariant=Sum_PI  TsampFilterVariant=InternalTs  TsampNgainVariant=Passthrough  TsampIntegralVariant=Passthrough  ExternalSaturationOutDataTypeStr=Inherit: Same as second input  aMode=0
  PI Controller for z axis : slpidlib/PID Controller  Commented=on  Controller=PI  Form=Parallel  TimeDomain=Continuous-time  UseExternalTs=off  SampleTime=-1  IntegratorMethod=Forward Euler  FilterMethod=Forward Euler  ControllerParametersSource=internal  P=PIController.z.P  I=PIController.z.I  UseKiTs=off  D=0  N=100  UseFilter=on  TunerSelectOption=Transfer Function Based (PID Tuner App)  InitialConditionSource=internal  InitialConditionForIntegrator=0  InitialConditionForFilter=0  DifferentiatorICPrevScaledInput=0  ExternalReset=none  TrackingMode=off  Kt=1  LimitOutput=off  SatLimitsSource=internal  UpperSaturationLimit=inf  LowerSaturationLimit=-inf  LinearizeAsGain=on  AntiWindupMode=none  Kb=1  POutMin=[]  POutMax=[]  IOutMin=[]  IOutMax=[]  DOutMin=[]  DOutMax=[]  NOutMin=[]  NOutMax=[]  SumOutMin=[]  SumOutMax=[]  SaturationOutMin=[]  SaturationOutMax=[]  PParamMin=[]  PParamMax=[]  IParamMin=[]  IParamMax=[]  DParamMin=[]  DParamMax=[]  NParamMin=[]  NParamMax=[]  KbParamMin=[]  KbParamMax=[]  KtParamMin=[]  KtParamMax=[]  KbOutMin=[]  KbOutMax=[]  KtOutMin=[]  KtOutMax=[]  IntegratorOutMin=[]  IntegratorOutMax=[]  FilterOutMin=[]  FilterOutMax=[]  SumI1OutMin=[]  SumI1OutMax=[]  SumI2OutMin=[]  SumI2OutMax=[]  SumI3OutMin=[]  SumI3OutMax=[]  SumI4OutMin=[]  SumI4OutMax=[]  SumDOutMin=[]  SumDOutMax=[]  DifferentiatorOutMin=[]  DifferentiatorOutMax=[]  FilterDiffOutCoefMin=[]  FilterDiffOutCoefMax=[]  ReciprocalOutMin=[]  ReciprocalOutMax=[]  SumDenOutMin=[]  SumDenOutMax=[]  SumNumOutMin=[]  SumNumOutMax=[]  DivideOutMin=[]  DivideOutMax=[]  UdiffTsProdOutMin=[]  UdiffTsProdOutMax=[]  NTsProdOutMin=[]  NTsProdOutMax=[]  UintegralTsProdOutMin=[]  UintegralTsProdOutMax=[]  UngainTsProdOutMin=[]  UngainTsProdOutMax=[]  IntegratorContinuousStateAttributes=''  IntegratorStateMustResolveToSignalObject=off  IntegratorRTWStateStorageClass=Auto  FilterContinuousStateAttributes=''  FilterStateMustResolveToSignalObject=off  FilterRTWStateStorageClass=Auto  ParallelPVariant=InternalParameters  IdealPVariant=Disabled  IVariant=InternalParameters  DVariant=Disabled  IntegratorVariant=Continuous  SatVariant=Disabled  AWVariant=Passthrough  PCopyVariant=Disabled  TRVariant=Disabled  FdbkBlocksVariant=Forward  IdealPFdbkVariant=Disabled  SatFdbkVariant=Disabled  DerivativeFilterVariant=Disabled  NVariant=Disabled  NCopyVariant=Disabled_SignalSpec  FilterICVariant=Disabled  IntegratorICVariant=InternalICs  ExternalResetVariant=Disabled  TRSumVariant=Passthrough  SumFdbkVariant=Disabled  SumVariant=Sum_PI  TsampFilterVariant=InternalTs  TsampNgainVariant=Passthrough  TsampIntegralVariant=Passthrough  ExternalSaturationOutDataTypeStr=Inherit: Same as second input  aMode=0
  Pilot commands storehouse : Subsystem
  Rotation Speed(TVC OFF)OK : Subsystem
  Rudder Saturation : Saturate  UpperLimit=Aactuator.rudder.AngleLimitUpper  LowerLimit=Aactuator.rudder.AngleLimitLower
  SB_deg3 : Goto  Commented=on  GotoTag=Autopilot_SB_deg
  Selector : Selector  InputPortWidth=3  IndexOptions=Index vector (dialog)  Indices=3  OutputSizes=1
  Selector1 : Selector  Commented=on  InputPortWidth=3  IndexOptions=Index vector (dialog)  Indices=3  OutputSizes=1
  Step : Step  Time=sysID_OBES.start_time  SampleTime=0
  Sum : Sum  Commented=on  Inputs=|++
  Sum1 : Sum  Inputs=|+-
  Sum2 : Sum  Commented=on  Inputs=|+-
  Sum3 : Sum  Commented=on  Inputs=|+-
  Sum4 : Sum  Inputs=|+-
  Switch : Switch  Commented=on  Criteria=u2 ~= 0  SaturateOnIntegerOverflow=off  InputSameDT=off
  Switch1 : Switch  Commented=on  Criteria=u2 ~= 0  SaturateOnIntegerOverflow=off  InputSameDT=off
  Switch2 : Switch  Criteria=u2 > Threshold  SaturateOnIntegerOverflow=off  InputSameDT=off
  TVC_lY Saturation : Saturate  UpperLimit=Aactuator.TVC_Z.AngleLimitUpper  LowerLimit=Aactuator.TVC_Z.AngleLimitLower
  TVC_lZ Saturation : Saturate  UpperLimit=Aactuator.TVC_Y.AngleLimitUpper  LowerLimit=Aactuator.TVC_Y.AngleLimitLower
  TVC_rY Saturation : Saturate  UpperLimit=Aactuator.TVC_Z.AngleLimitUpper  LowerLimit=Aactuator.TVC_Z.AngleLimitLower
  TVC_rZ Saturation : Saturate  UpperLimit=Aactuator.TVC_Y.AngleLimitUpper  LowerLimit=Aactuator.TVC_Y.AngleLimitLower
  Terminator1 : Terminator  Commented=on
  Terminator2 : Terminator  Commented=on
  Terminator3 : Terminator  Commented=on
  Transfer Fcn1 : TransferFcn  Commented=on  Numerator=[25]  Denominator=[1 10 25]
  Transfer Fcn2 : TransferFcn  Numerator=[25]  Denominator=[1 10 25]
  Transfer Fcn3 : TransferFcn  Numerator=[25]  Denominator=[1 10 25]
  Transfer Fcn4 : TransferFcn  Commented=on  Numerator=[25]  Denominator=[1 10 25]
  Vehicle : Subsystem
  beta_c : Constant  Commented=on  Value=0
  pqr NDI Controller : Subsystem  VariantControl=TVC ON
  sysID_Onboard_Excitation_System : Subsystem
  thrust1 : Constant  Value=IC.thrust_lbf
  μαβ NDI Controller : Subsystem
  庭宇 6.3節短場降落(模擬秒數設定:inf) : Subsystem  Tag=STV Subsys  Commented=on  LoadFcn=sigbuilder_block('load');  StartFcn=sigbuilder_block('start');  StopFcn=sigbuilder_block('stop');  ClipboardFcn=sigbuilder_block('clipboard');  mask(Sigbuilder block){tuvar=[0:10]}
      mask help: Simulink:masks:SigbuilderBlock_MD
      mask init:
      | if ~strcmp(get_param(bdroot(gcbh),'SimulationStatus'),'stopped') tuvar = sigbuilder_block('maskInit'); end
      settings: CopyFcn=sigbuilder_block('copy');  DeleteFcn=sigbuilder_block('delete');  ModelCloseFcn=sigbuilder_block('modelClose');  PreSaveFcn=sigbuilder_block('preSave');  PauseFcn=sigbuilder_block('pause');  ContinueFcn=sigbuilder_block('continue');  NameChangeFcn=sigbuilder_block('namechange');  OpenFcn=sigbuilder_block('open',[6 30 1428 680.25 ]);  CloseFcn=sigbuilder_block('close');
      mask Display: plot(0, 0, 100, 100,[2, 2, 32, 32, 2], [68, 8, 8, 68, 68],[32, 2], [38, 38], [32, 19, 2],[53, 60, 44], [32, 17, 17, 2],[16, 16, 31, 31]);txt = getActiveGroup(gcbh);text(2, 100, txt,'verticalAlignment', 'top');
  落葉飄完整版(碩論6.7)1 : Subsystem  Tag=STV Subsys  LoadFcn=sigbuilder_block('load');  StartFcn=sigbuilder_block('start');  StopFcn=sigbuilder_block('stop');  ClipboardFcn=sigbuilder_block('clipboard');  mask(Sigbuilder block){tuvar=[0:10]}
      mask help: Simulink:masks:SigbuilderBlock_MD
      mask init:
      | if ~strcmp(get_param(bdroot(gcbh),'SimulationStatus'),'stopped') tuvar = sigbuilder_block('maskInit'); end
      settings: CopyFcn=sigbuilder_block('copy');  DeleteFcn=sigbuilder_block('delete');  ModelCloseFcn=sigbuilder_block('modelClose');  PreSaveFcn=sigbuilder_block('preSave');  PauseFcn=sigbuilder_block('pause');  ContinueFcn=sigbuilder_block('continue');  NameChangeFcn=sigbuilder_block('namechange');  OpenFcn=sigbuilder_block('open',[6 30 1428 680.25 ]);  CloseFcn=sigbuilder_block('close');
      mask Display: plot(0, 0, 100, 100,[2, 2, 32, 32, 2], [68, 8, 8, 68, 68],[32, 2], [38, 38], [32, 19, 2],[53, 60, 44], [32, 17, 17, 2],[16, 16, 31, 31]);txt = getActiveGroup(gcbh);text(2, 100, txt,'verticalAlignment', 'top');
  Plant_Data : Outport
  Env_Data : Outport  Port=2
  wires:
  Aerodynamic1/3(aero_control fast G) -> [NDI_aero_control_fast_G]
  PI Controller for yaw/1 -> Mux1/3
  Demux3/2 -> PI Controller for pitch/1
  PI Controller for roll/1 -> Mux1/1
  Bus Selector1/2 -> Mux16/2  "<q>"
  Demux3/3 -> PI Controller for yaw/1
  In Bus Element1/1 -> Vehicle/5(EnvData)
  Bus Selector1/3 -> Mux16/3  "<r>"
  [SB_deg] -> Aerodynamic1/1(SB (deg))
  Bus Selector1/1 -> Mux16/1  "<p>"
  [SB_deg] -> Vehicle/3(" SB_deg")
  Aerodynamic1/2(aero_control M) -> [NDI_aero_control_M]
  Mux1/1 -> pqr NDI Controller/3(pqr dot desire)  "pqr dot desire"
  Aerodynamic1/1(aero_control F) -> [NDI_aero_control_F]
  PI Controller for pitch/1 -> Mux1/2
  In Bus Element3/1 -> Env_Data/1
  Demux3/1 -> PI Controller for roll/1
  PI Controller for beta/1 -> Mux6/3
  Mux6/1 -> μαβ NDI Controller/2(μαβ dot desire)  "mu alpha beta dot desire"
  Bus Selector4/3 -> Mux18/3  "<beta>"
  PI Controller for mu/1 -> Mux6/1
  Bus Selector4/1 -> Mux18/1  "<mu>"
  Bus Selector4/2 -> Mux18/2  "<alpha>"
  Mux18/1 -> Sum4/2
  Demux6/1 -> PI Controller for mu/1
  Transfer Fcn3/1 -> Mux5/3  "beta_c"
  PI Controller for alpha/1 -> Mux6/2
  μαβ NDI Controller/1(pc) -> Mux2/1
  [LGxyz] -> μαβ NDI Controller/3(LGxyz)
  [NDI_aero_control_F] -> μαβ NDI Controller/1(aero F)
  μαβ NDI Controller/5(Y) -> Mux11/2
  Transfer Fcn2/1 -> Mux5/1  "mu_c"
  μαβ NDI Controller/3(rc) -> Mux2/3
  μαβ NDI Controller/2(qc) -> Mux2/2
  μαβ NDI Controller/4(D) -> Mux11/1
  Demux6/2 -> PI Controller for alpha/1
  Demux6/3 -> PI Controller for beta/1
  μαβ NDI Controller/6(L) -> Mux11/3
  Bus Creator2/1 -> Vehicle/2(fcs_cmd)
  Bus Creator/1 -> Vehicle/1(fadec_cmd)
  Manual Switch1/1 -> Bus Creator/1  "thrust"
  thrust1/1 -> Manual Switch/1  "thrust"
  Elevator Saturation1/1 -> Bus Creator2/3  "right elevator"
  Elevator Saturation/1 -> Bus Creator2/4  "left elevator"
  Aileron Saturation1/1 -> Bus Creator2/2  "left aileron"
  Aileron Saturation/1 -> Bus Creator2/1  "right aileron"
  Rudder Saturation/1 -> Bus Creator2/5  "rudder"
  TVC_rZ Saturation/1 -> Bus Creator/2  "TVC_ry"
  TVC_rY Saturation/1 -> Bus Creator/3  "TVC_rz"
  TVC_lZ Saturation/1 -> Bus Creator/4  "TVC_ly"
  TVC_lY Saturation/1 -> Bus Creator/5  "TVC_lz"
  [LG_down] -> Vehicle/4(LG_cmd)
  Rotation Speed(TVC OFF)OK/1(Output) -> Manual Switch5/2
  Mux7/1 -> Landing_Control/2(mu_alpha_beta)  "mu alpha beta command (rad)"
  Demux/3 -> Sum/1  "h_ft"
  Aerodynamic2/1(aero_control F) -> Iteration Algorithm V chi gamma/2(aero F)
  From4/1 -> Aerodynamic2/1(SB (deg))
  From5/1 -> Iteration Algorithm V chi gamma/5(LGxyz)
  Gain/1 -> Mux10/2  "z_ft"
  Transfer Fcn4/1 -> Mux3/2
  Sum3/1 -> Demux5/1  "yz err"
  Bus Selector5/1 -> Switch/2  "<Nose_WOW>"
  Switch/1 -> SB_deg3/1
  Bus Selector/1 -> Mux12/1  "<epos>"
  Aerodynamic2/4(LEF) -> Terminator3/1
  Aerodynamic2/2(aero_control M) -> Terminator1/1
  Constant/1 -> Sum/2
  Aerodynamic2/3(aero_control fast G) -> Terminator2/1
  PI Controller for Vt/1 -> Mux4/1
  Bus Creator1/1 -> Aerodynamic2/3(AirData)
  Bus Selector3/3 -> Mux17/3  "<gamma>"
  IC/1 -> Iteration Algorithm V chi gamma/1(alpha_c)  "α_c (rad)"
  Iteration Algorithm Y Z/2(gamma_c) -> Transfer Fcn1/1
  Iteration Algorithm V chi gamma/4(beta_command) -> Bus Creator1/1, Mux7/3  "beta"
  Demux5/1 -> PI Controller for y axis/1
  Mux4/1 -> Iteration Algorithm V chi gamma/3(Vt,chi,gamma dot desire)  "Vt chi gamma dot desire"
  Iteration Algorithm Y Z/1(chi_c) -> Transfer Fcn4/1
  Transfer Fcn1/1 -> Mux3/3
  Iteration Algorithm V chi gamma/2(mu_command) -> Mux7/1  "mu_c"
  Demux1/1 -> PI Controller for Vt/1
  Sum/1 -> Gain/1
  Mux12/1 -> Sum3/2
  From/1 -> Aerodynamic2/2(PlantData)
  Bus Selector3/1 -> Mux17/1  "<Vt>"
  Demux/4 -> Switch/3  "SB_deg"
  beta_c/1 -> Iteration Algorithm V chi gamma/4(beta_cmd)
  Landing_Control/1(thrust_command) -> Manual Switch1/2  "thrust"
  Mux9/1 -> Iteration Algorithm Y Z/2(Ydot,Zdot des)  "y z dot desire"
  Landing_Control/2(mu_alpha_beta_command) -> Manual Switch2/2
  Demux/2 -> Mux10/1  "y_ft"
  Iteration Algorithm V chi gamma/1(thrust_command) -> Landing_Control/1(thrust)  "thrust"
  Bus Selector3/2 -> Mux17/2  "<chi>"
  Constant1/1 -> Switch/1
  PI Controller for y axis/1 -> Mux9/1
  Bus Selector/2 -> Mux12/2  "<altitude>"
  Demux/1 -> Switch1/3  "Vt"
  PI Controller for z axis/1 -> Mux9/2
  Mux17/1 -> Sum2/2
  Demux5/2 -> PI Controller for z axis/1
  Manual Switch/1 -> Manual Switch1/1  "thrust"
  Mux5/1 -> Manual Switch2/1  "mu alpha beta command (rad)"
  Manual Switch3/1 -> [LG_down]  "mu alpha beta command (rad)"
  Manual Switch4/1 -> [SB_deg]  "mu alpha beta command (rad)"
  [Autopilot_SB_deg] -> Manual Switch4/2
  [Autopilot_LG_down] -> Manual Switch3/2
  Bus Selector2/1 -> Switch1/1  "<Vt>"
  Switch1/1 -> Iteration Algorithm Y Z/1(Vc), Mux3/1
  Logical Operator/1 -> Switch1/2
  Bus Selector6/1 -> Logical Operator/1  "<RightMain_WOW>"
  Bus Selector6/2 -> Logical Operator/2  "<LeftMain_WOW>"
  Mux13/1 -> Goto/1
  Demux/5 -> Mux13/1, Mux13/3, Mux13/2  "LG_down"
  In Bus Element2/1 -> Selector/1
  Selector/1 -> μαβ NDI Controller/4(gravity)
  In Bus Element/1 -> Selector1/1
  Selector1/1 -> Iteration Algorithm V chi gamma/6(gravity)
  sysID_Onboard_Excitation_System/9(rudder) -> Add8/2
  sysID_Onboard_Excitation_System/8(left_elevator) -> Add7/2
  sysID_Onboard_Excitation_System/7(right_elevator) -> Add6/2
  sysID_Onboard_Excitation_System/6(left_aileron) -> Add5/2
  sysID_Onboard_Excitation_System/5(right_aileron) -> Add4/2
  sysID_Onboard_Excitation_System/4(TVC_lz) -> Add3/2
  sysID_Onboard_Excitation_System/3(TVC_ly) -> Add2/2
  sysID_Onboard_Excitation_System/2(TVC_rz) -> Add1/2
  sysID_Onboard_Excitation_System/1(TVC_ry) -> Add/2
  pqr NDI Controller/3("TVC_ly ") -> Add2/1  "TVC_ly"
  pqr NDI Controller/1("TVC_ry ") -> Add/1  "TVC_ry"
  Add/1 -> TVC_rZ Saturation/1
  Add8/1 -> Rudder Saturation/1
  Add7/1 -> Elevator Saturation/1
  Add6/1 -> Elevator Saturation1/1
  Add5/1 -> Aileron Saturation1/1
  Add4/1 -> Aileron Saturation/1
  Add3/1 -> TVC_lY Saturation/1
  Add1/1 -> TVC_rY Saturation/1
  Add2/1 -> TVC_lZ Saturation/1
  Step/1 -> Switch2/1
  Switch2/1 -> sysID_Onboard_Excitation_System/1(Enable)
  Constant7/1 -> Switch2/3
  Constant8/1 -> Switch2/2
  pqr NDI Controller/7(right_elevator) -> Add6/1  "right elevator"
  pqr NDI Controller/8(left_elevator) -> Add7/1  "left elevator"
  Aerodynamic1/4(LEF) -> [LEF]
  Bus Creator3/1 -> Vehicle/6(LogDataBus)
  Demux1/2 -> PI Controller for chi/1
  Demux1/3 -> PI Controller for gamma/1
  [cmd_pqr] -> Bus Creator3/4  "cmd_pqr"
  [cmd_mu_alpha_beta] -> Bus Creator3/3  "cmd_mu_alpha_beta"
  [cmd_Vt_chi_gamma] -> Bus Creator3/2  "cmd_Vt_chi_gamma"
  [LEF] -> Bus Creator2/6  "LEF"
  [DYL] -> Bus Creator3/5  "drag_sideForce_lift"
  [cmd_yz] -> Bus Creator3/1  "cmd_yz"
  落葉飄完整版(碩論6.7)1/1(thrust) -> Manual Switch/2
  Iteration Algorithm V chi gamma/3(alpha_command) -> IC/1, Bus Creator1/2, Mux7/2  "alpha"
  Manual Switch2/1 -> Sum4/1, [cmd_mu_alpha_beta]  "mu alpha beta command (rad)"
  Manual Switch5/1 -> Sum1/1, [cmd_pqr]
  Mux10/1 -> Sum3/1, Goto8/1  "yz command"
  Mux11/1 -> [DYL]  "Drag  Side Force Lift"
  Mux16/1 -> pqr NDI Controller/4(p q r), Sum1/2
  Mux2/1 -> Rotation Speed(TVC OFF)OK/1(pqr command), Manual Switch5/1  "pqr command (rad/s)"
  Mux3/1 -> Sum2/1, Goto1/1  "Vt chi gamma command"
  PI Controller for chi/1 -> Mux4/2
  PI Controller for gamma/1 -> Mux4/3
  Sum1/1 -> Demux3/1  "pqr err"
  Sum2/1 -> Demux1/1  "Vt chi gamma err"
  Sum4/1 -> Demux6/1  "mu alpha beta err"
  [NDI_aero_control_M] -> pqr NDI Controller/1(coef M)
  [NDI_aero_control_fast_G] -> pqr NDI Controller/2(control g)
  Vehicle/1(PlantData) -> Aerodynamic1/2(PlantData), Aerodynamic1/3(AirData), Bus Selector1/1, μαβ NDI Controller/5(AirData), μαβ NDI Controller/6(PlantData), Bus Selector4/1, Landing_Control/3(PlantData), Goto2/1, Iteration Algorithm V chi gamma/7(AirData), Iteration Algorithm V chi gamma/8(PlantData), Bus Selector2/1, Bus Selector6/1, Bus Selector5/1, Bus Selector/1, Bus Selector3/1, Rotation Speed(TVC OFF)OK/2(PlantData), pqr NDI Controller/5(PlantData), Plant_Data/1
  庭宇 6.3節短場降落(模擬秒數設定:inf)/3(h_ft) -> Mux19/3  "h_ft"
  庭宇 6.3節短場降落(模擬秒數設定:inf)/1(Vt) -> Mux19/1  "Vt"
  庭宇 6.3節短場降落(模擬秒數設定:inf)/4(SB_deg) -> Mux19/4  "SB_deg"
  Multiport Switch/1 -> Demux/1
  Mux19/1 -> Multiport Switch/4
  Mux8/1 -> Multiport Switch/3
  庭宇 6.3節短場降落(模擬秒數設定:inf)/2(y_ft) -> Mux19/2  "y_ft"
  庭宇 6.3節短場降落(模擬秒數設定:inf)/5(LandingGear_down) -> Mux19/5  "LG_down"
  Mux15/1 -> Multiport Switch/2
  Constant14/1 -> Multiport Switch/1
  Constant4/1 -> Mux8/3  "h_ft"
  Constant5/1 -> Mux8/4  "SB_deg"
  Constant3/1 -> Mux8/2  "y_ft"
  Constant2/1 -> Mux8/1  "Vt"
  Constant6/1 -> Mux8/5  "LG_down"
  Constant13/1 -> Mux15/5  "LG_down"
  Constant9/1 -> Mux15/1  "Vt"
  Constant10/1 -> Mux15/2  "y_ft"
  Constant12/1 -> Mux15/4  "SB_deg"
  Constant11/1 -> Mux15/3  "h_ft"
  Gain1/1 -> Add1/1
  Gain2/1 -> Add3/1
  Gain3/1 -> Add4/1
  Gain4/1 -> Add5/1
  Gain5/1 -> Add8/1
  pqr NDI Controller/2(TVC_rz) -> Gain1/1  "TVC_rz"
  pqr NDI Controller/4("TVC_lz ") -> Gain2/1  "TVC_lz"
  pqr NDI Controller/5(right_aileron) -> Gain3/1  "right aileron"
  pqr NDI Controller/6(left_aileron) -> Gain4/1  "left aileron"
  pqr NDI Controller/9(rudder) -> Gain5/1  "rudder"
  Manual Switch8/1 -> Transfer Fcn2/1  "mu alpha beta command (rad)"
  Manual Switch7/1 -> Mux5/2  "mu alpha beta command (rad)"
  Manual Switch6/1 -> Transfer Fcn3/1  "mu alpha beta command (rad)"
  落葉飄完整版(碩論6.7)1/4(beta) -> Angle Conversion5/1
  落葉飄完整版(碩論6.7)1/3(alpha) -> Angle Conversion4/1
  落葉飄完整版(碩論6.7)1/2(mu) -> Angle Conversion3/1
  Constant16/1 -> Manual Switch8/1
  Constant15/1 -> Manual Switch7/1
  Constant17/1 -> Manual Switch6/1
  落葉飄完整版(碩論6.7)1/5(speed brake) -> Manual Switch9/2
  Manual Switch9/1 -> Manual Switch4/1
  Mux14/1 -> Manual Switch3/1
  落葉飄完整版(碩論6.7)1/6(LandingGear_down) -> Manual Switch10/2
  Manual Switch10/1 -> Mux14/3, Mux14/1, Mux14/2  "mu alpha beta command (rad)"
  Constant18/1 -> Manual Switch9/1
  Constant19/1 -> Manual Switch10/1
  Angle Conversion3/1 -> Manual Switch8/2
  Angle Conversion4/1 -> Manual Switch7/2  "alpha_c"
  Angle Conversion5/1 -> Manual Switch6/2
